simulink model "sim_1"  (R2022b)
settings: Solver=VariableStepAuto  StartTime=0.0  StopTime=60  RelTol=1e-3
settings Model: Creator=mrxmi  LastModifiedBy=mrxmi

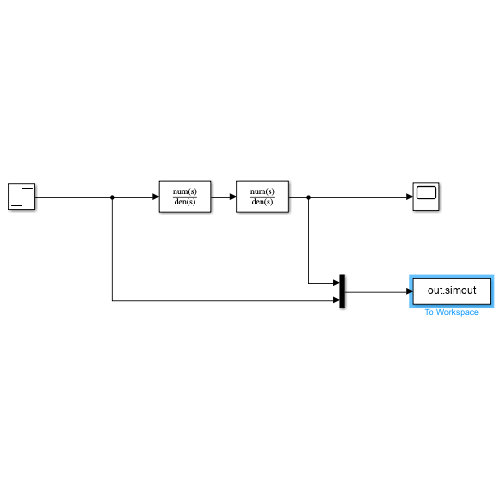
[thumbnail: Simulink's stored preview of the top-level diagram]
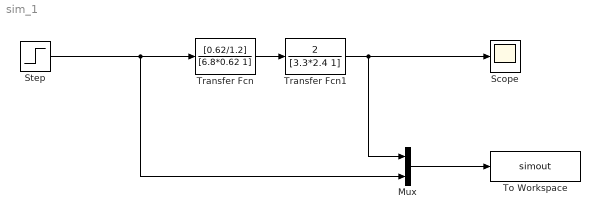
== system sim_1 ==
  Mux : Mux  Inputs=2
  Scope : Scope
  Step : Step  SampleTime=0
  To Workspace : ToWorkspace  VariableName=simout  SaveFormat=Structure With Time  SampleTime=-1
  Transfer Fcn : TransferFcn  Numerator=[0.62/1.2]  Denominator=[6.8*0.62 1]
  Transfer Fcn1 : TransferFcn  Numerator=[2]  Denominator=[3.3*2.4 1]
  wires:
  Transfer Fcn/1 -> Transfer Fcn1/1
  Transfer Fcn1/1 -> Mux/1, Scope/1
  Step/1 -> Mux/2, Transfer Fcn/1
  Mux/1 -> To Workspace/1
